simulink model "Question7"  (R2020a)
settings: Solver=VariableStepAuto  StartTime=0.0  StopTime=10.0  RelTol=1e-3
settings Model: Creator=aishw  LastModifiedBy=aishw

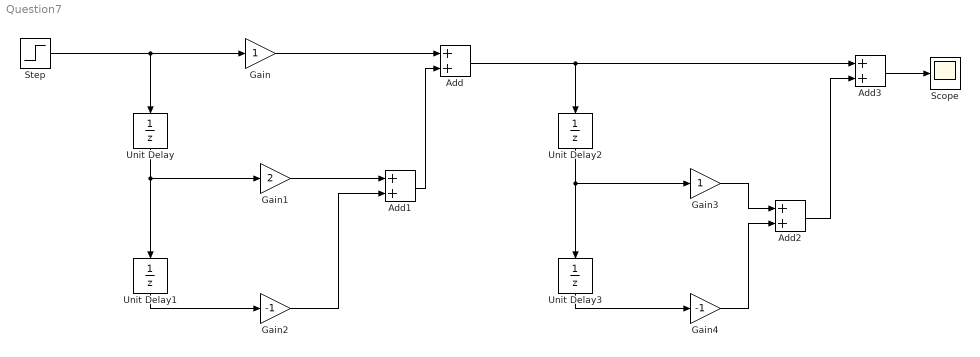
== system Question7 ==
  Add{,1..3} (4 alike) : Sum
  Gain : Gain
  Gain1 : Gain  Gain=2
  Gain2 : Gain  Gain=-1
  Gain3 : Gain
  Gain4 : Gain  Gain=-1
  Scope : Scope
  Step : Step  SampleTime=0
  Unit Delay{,1..3} (4 alike) : UnitDelay  SampleTime=-1  HasFrameUpgradeWarning=on
  wires:
  Step/1 -> Unit Delay/1, Gain/1
  Unit Delay/1 -> Unit Delay1/1, Gain1/1
  Unit Delay1/1 -> Gain2/1
  Gain2/1 -> Add1/2
  Gain1/1 -> Add1/1
  Add1/1 -> Add/2
  Gain/1 -> Add/1
  Add/1 -> Unit Delay2/1, Add3/1
  Unit Delay2/1 -> Gain3/1, Unit Delay3/1
  Unit Delay3/1 -> Gain4/1
  Gain4/1 -> Add2/2
  Gain3/1 -> Add2/1
  Add2/1 -> Add3/2
  Add3/1 -> Scope/1
